simulink subsystem "RoboRio_Controls_sub"  (R2023b)
settings: Solver=VariableStepAuto  StartTime=0.0  StopTime=10.0  RelTol=1e-3
undefined symbols (not defined in the file): Odometry_IC_X, Odometry_IC_Y
libraries: Autonomous_lib x1, simulink_extras x1, Disabled_lib x1, Teleop_lib x1, Test_lib x1
settings Model: Creator=USER  LastModifiedBy=ander

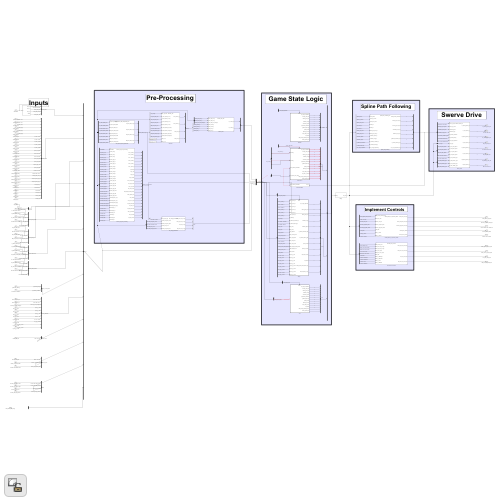
[thumbnail: Simulink's stored preview of the top-level diagram]
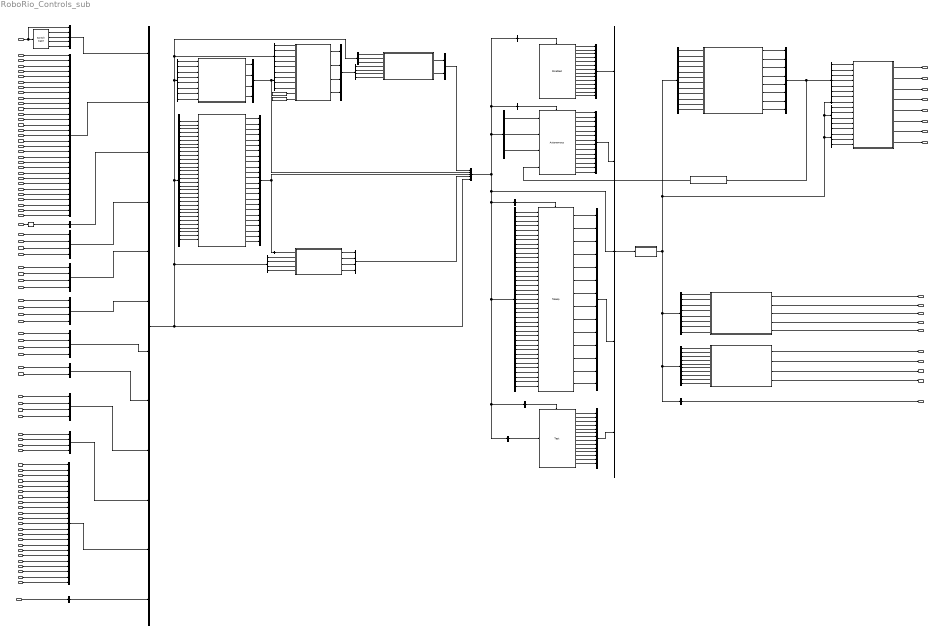
== system RoboRio_Controls_sub ==
  note: Game State Logic
  note: Swerve Drive
  note: Inputs
  note: Pre-Processing
  note: Spline Path
      | Following
  note: Implement Controls
  GameState : Inport
  Joystick_Left_X : Inport  Port=2
  Joystick_Left_Y : Inport  Port=3
  Joystick_Left_Z : Inport  Port=4
  Joystick_Right_X : Inport  Port=5
  Joystick_Right_Y : Inport  Port=6
  Joystick_Right_Z : Inport  Port=7
  Joystick_Left_B1 : Inport  Port=8
  Joystick_Left_B2 : Inport  Port=9
  Joystick_Left_B3 : Inport  Port=10
  Joystick_Left_B4 : Inport  Port=11
  Joystick_Left_B7 : Inport  Port=12
  Joystick_Left_B8 : Inport  Port=13
  Joystick_Left_B10 : Inport  Port=14
  Joystick_Right_B1 : Inport  Port=15
  Joystick_Right_B2 : Inport  Port=16
  Joystick_Right_B3 : Inport  Port=17
  Joystick_Right_B4 : Inport  Port=18
  Joystick_Right_POV : Inport  Port=19
  Joystick_Right_B7 : Inport  Port=20
  Joystick_Right_B8 : Inport  Port=21
  Joystick_Right_B10 : Inport  Port=22
  Gamepad_Stick_Left_X : Inport  Port=23
  Gamepad_Stick_Left_Y : Inport  Port=24
  Gamepad_Stick_Right_X : Inport  Port=25
  Gamepad_Stick_Right_Y : Inport  Port=26
  Gamepad_B1_A : Inport  Port=27
  Gamepad_B3_X : Inport  Port=28
  Gamepad_LB : Inport  Port=29
  Gamepad_LT : Inport  Port=30
  Gamepad_RB : Inport  Port=31
  Gamepad_RT : Inport  Port=32
  Gyro_Angle : Inport  Port=33
  FL_Drive_Motor_Speed : Inport  Port=34
  FR_Drive_Motor_Speed : Inport  Port=35
  BL_Drive_Motor_Speed : Inport  Port=36
  BR_Drive_Motor_Speed : Inport  Port=37
  FL_Drive_Motor_Rev : Inport  Port=38
  FR_Drive_Motor_Rev : Inport  Port=39
  BL_Drive_Motor_Rev : Inport  Port=40
  BR_Drive_Motor_Rev : Inport  Port=41
  FL_Steer_Module_Rev : Inport  Port=42
  FR_Steer_Module_Rev : Inport  Port=43
  BL_Steer_Module_Rev : Inport  Port=44
  BR_Steer_Module_Rev : Inport  Port=45
  FL_Steer_Module_Offset : Inport  Port=46
  FR_Steer_Module_Offset : Inport  Port=47
  BL_Steer_Module_Offset : Inport  Port=48
  BR_Steer_Module_Offset : Inport  Port=49
  Is_Absolute_Steering : Inport  Port=50
  Is_Absolute_Translation : Inport  Port=51
  Intake_TOF_Dist : Inport  Port=52
  Shooter_TOF_Dist : Inport  Port=53
  Shooter_Left_Motor_RPM : Inport  Port=54
  Shooter_Right_Motor_RPM : Inport  Port=55
  Encoder_Revs_Back_Lower : Inport  Port=56
  Encoder_Revs_Back_Upper : Inport  Port=57
  Encoder_Revs_Front : Inport  Port=58
  Encoder_Revs_Ball_Screw : Inport  Port=59
  Photon_Est_Pose_X : Inport  Port=60
  Photon_Est_Pose_Y : Inport  Port=61
  Photon_Est_Pose_Ambiguity : Inport  Port=62
  AT_Tag_4_Yaw : Inport  Port=63
  AT_Tag_5_Yaw : Inport  Port=64
  AT_Tag_6_Yaw : Inport  Port=65
  AT_Tag_7_Yaw : Inport  Port=66
  AT_Tag_11_Yaw : Inport  Port=67
  AT_Tag_12_Yaw : Inport  Port=68
  AT_Tag_13_Yaw : Inport  Port=69
  AT_Tag_14_Yaw : Inport  Port=70
  AT_Tag_15_Yaw : Inport  Port=71
  AT_Tag_16_Yaw : Inport  Port=72
  AT_Tag_4_Found : Inport  Port=73
  AT_Tag_5_Found : Inport  Port=74
  AT_Tag_6_Found : Inport  Port=75
  AT_Tag_7_Found : Inport  Port=76
  Line_Sensor_TOF_Range : Inport  Port=77
  AT_Tag_11_Found : Inport  Port=78
  AT_Tag_12_Found : Inport  Port=79
  AT_Tag_13_Found : Inport  Port=80
  AT_Tag_14_Found : Inport  Port=81
  AT_Tag_15_Found : Inport  Port=82
  AT_Tag_16_Found : Inport  Port=83
  Arm_Length_Calculation : Subsystem  ReferencedSubsystem=Arm_Length_Calculation
  Autonomous : Autonomous_lib/Autonomous  SystemSampleTime=-1  VariantActivationTime=update diagram  AllowFlexibleInterface=on  Latency=0  AutoFrameSizeCalculation=off
  Bus Creator : BusCreator  Inputs=5
  Bus Creator{1..2,4,12} (4 alike) : BusCreator  Inputs=14
  Bus Creator10 : BusCreator  Inputs=2
  Bus Creator11 : BusCreator  Inputs=12
  Bus Creator13 : BusCreator  Inputs=8
  Bus Creator{7..9,14..16,21..23} (9 alike) : BusCreator  Inputs=4
  Bus Creator17 : BusCreator  Inputs=5
  Bus Creator18 : BusCreator  Inputs=23
  Bus Creator19 : BusCreator  Inputs=2
  Bus Creator24 : BusCreator  Inputs=24
  Bus Creator25 : BusCreator  Inputs=1
  Bus Creator3 : BusCreator  Inputs=5
  Bus Creator5 : BusCreator  Inputs=31
  Bus Creator6 : BusCreator  Inputs=1
  Bus Selector : BusSelector  OutputSignals=Steering_Abs_Cmd_SPF,Steering_Rel_Cmd_SPF,Translation_Speed_SPF,Translation_Angle_SPF,Is_Absolute_Translation_SPF,Is_Absolute_Steering_SPF,Gyro_Angle_Adjustment_SPF
  Bus Selector1 : BusSelector  OutputSignals=Odom_Position_X,Odom_Position_Y,Odom_Delta_X,Odom_Delta_Y
  Bus Selector10 : BusSelector  OutputSignals=PreProcessing.Inputs.IMU_Sensor.Gyro_Angle
  Bus Selector11 : BusSelector  OutputSignals=State_Request_Arm,PreProcessing.Arms.Back_Lower_Arm_Length,PreProcessing.Arms.Back_Upper_Arm_Length,PreProcessing.Arms.Front_Arm_Length,PreProcessing.Arms.Ball_Screw_Arm_Length,Test_Mode,PreProcessing.Human_Inputs.Test_DC_BackUpper,PreProcessing.Human_Inputs.Test_DC_BackLower,PreProcessing.Human_Inputs.Test_DC_Front,PreProcessing.Human_Inputs.Test_DC_BallScrew
  Bus Selector12 : BusSelector  OutputSignals=Human_Inputs.Chain_Hook
  Bus Selector13 : BusSelector  OutputSignals=Game_States.GameState,Human_Inputs.Joystick_Left_X,Human_Inputs.Joystick_Left_Y,Human_Inputs.Joystick_Left_Z,Human_Inputs.Joystick_Right_X,Human_Inputs.Joystick_Right_Y,Human_Inputs.Joystick_Right_Z,Human_Inputs.Joystick_Left_B1,Human_Inputs.Joystick_Left_B2,Human_Inputs.Joystick_Left_B3,Human_Inputs.Joystick_Left_B4,Human_Inputs.Joystick_Left_B7,Human_Inputs.Joystick_Left_B8,Human_Inputs.Joystick_Left_B10,Human_Inputs.Joystick_Right_B1,Human_Inputs.Joystick_Right_B2,Human_Inputs.Joystick_Right_B3,Human_Inputs.Joystick_Right_B4,Human_Inputs.Joystick_Right_POV,Human_Inputs.Joystick_Right_B7,Human_Inputs.Joystick_Right_B8,Human_Inputs.Joystick_Right_B10,Human_Inputs.Gamepad_Stick_Left_X,Human_Inputs.Gamepad_Stick_Left_Y,Human_Inputs.Gamepad_Stick_Right_X,Human_Inputs.Gamepad_Stick_Right_Y,Human_Inputs.Gamepad_B1_A,Human_Inputs.Gamepad_B3_X,Human_Inputs.Gamepad_LB,Human_Inputs.Gamepad_LT,Human_Inputs.Gamepad_RB,Human_Inputs.Gamepad_RT
  Bus Selector14 : BusSelector  OutputSignals=Arm_Dist_Cal_Flag
  Bus Selector15 : BusSelector  OutputSignals=Chain_DutyCycle
  Bus Selector2 : BusSelector  OutputSignals=Inputs.Game_States.Game_State_Teleop
  Bus Selector3 : BusSelector  OutputSignals=Photon_Estimates.Photon_Est_Pose_X,Photon_Estimates.Photon_Est_Pose_Y,Photon_Estimates.Photon_Est_Pose_Ambiguity
  Bus Selector4 : BusSelector  OutputSignals=Inputs.Game_States.Game_State_Auto
  Bus Selector40 : BusSelector  OutputSignals=IMU_Sensor.Gyro_Angle,Drive_Motor_Revs.FL_Drive_Motor_Rev,Drive_Motor_Revs.FR_Drive_Motor_Rev,Drive_Motor_Revs.BL_Drive_Motor_Rev,Drive_Motor_Revs.BR_Drive_Motor_Rev
  Bus Selector41 : BusSelector  OutputSignals=Human_Inputs.Drive_Joystick_X,Human_Inputs.Drive_Joystick_Y,Human_Inputs.Drive_Joystick_Z,Human_Inputs.Steer_Joystick_X,Human_Inputs.Steer_Joystick_Y,Human_Inputs.Steer_Joystick_Z,Human_Inputs.Is_Boosting,Inputs.Motion_Control_Modes.Is_Absolute_Translation,Inputs.Motion_Control_Modes.Is_Absolute_Steering,Human_Inputs.Align_Trap,Human_Inputs.Align_Amp,Human_Inputs.Align_Speaker,Human_Inputs.Face_Toward_Driver,Human_Inputs.Face_Right_Driver,Human_Inputs.Face_Left_Driver,Human_Inputs.Face_Away_Driver,Human_Inputs.State_Request_Intake_Shooter,Human_Inputs.State_Request_Arm,Human_Inputs.Chain_Hook,Inputs.Photon_Estimates.AT_Tag_4_Yaw,Inputs.Photon_Estimates.AT_Tag_5_Yaw,Inputs.Photon_Estimates.AT_Tag_6_Yaw,Inputs.Photon_Estimates.AT_Tag_7_Yaw,Inputs.Photon_Estimates.AT_Tag_11_Yaw,Inputs.Photon_Estimates.AT_Tag_12_Yaw,Inputs.Photon_Estimates.AT_Tag_13_Yaw,Inputs.Photon_Estimates.AT_Tag_14_Yaw,Inputs.Photon_Estimates.AT_Tag_15_Yaw,Inputs.Photon_Estimates.AT_Tag_16_Yaw,Inputs.Photon_Estimates.AT_Tag_4_Found,Inputs.Photon_Estimates.AT_Tag_5_Found,Inputs.Photon_Estimates.AT_Tag_6_Found,Inputs.Photon_Estimates.AT_Tag_7_Found,Inputs.Photon_Estimates.AT_Tag_11_Found,Inputs.Photon_Estimates.AT_Tag_12_Found,Inputs.Photon_Estimates.AT_Tag_13_Found,Inputs.Photon_Estimates.AT_Tag_14_Found,Inputs.Photon_Estimates.AT_Tag_15_Found,Inputs.Photon_Estimates.AT_Tag_16_Found
  Bus Selector5 : BusSelector  OutputSignals=State_Request_Intake_Shooter,PreProcessing.Inputs.Intake_and_Shooter.Intake_TOF_Dist,PreProcessing.Inputs.Intake_and_Shooter.Shooter_TOF_Dist,PreProcessing.Inputs.Intake_and_Shooter.Shooter_Left_Motor_RPM,PreProcessing.Inputs.Intake_and_Shooter.Shooter_Right_Motor_RPM,Test_Mode,PreProcessing.Human_Inputs.Test_DC_Intake,PreProcessing.Human_Inputs.Test_DC_Shooter
  Bus Selector50 : BusSelector  OutputSignals=PreProcessing.Inputs.Drive_Motor_Speeds.FL_Drive_Motor_Speed,PreProcessing.Inputs.Drive_Motor_Speeds.FR_Drive_Motor_Speed,PreProcessing.Inputs.Drive_Motor_Speeds.BL_Drive_Motor_Speed,PreProcessing.Inputs.Drive_Motor_Speeds.BR_Drive_Motor_Speed
  Bus Selector52 : BusSelector  OutputSignals=PreProcessing.Steer_Module_Angles.FL_Steer_Module_Angle,PreProcessing.Steer_Module_Angles.FR_Steer_Module_Angle,PreProcessing.Steer_Module_Angles.BL_Steer_Module_Angle,PreProcessing.Steer_Module_Angles.BR_Steer_Module_Angle
  Bus Selector57 : BusSelector  OutputSignals=Steer_Module_Revs.FL_Steer_Module_Rev,Steer_Module_Offsets.FL_Steer_Module_Offset,Steer_Module_Revs.FR_Steer_Module_Rev,Steer_Module_Offsets.FR_Steer_Module_Offset,Steer_Module_Revs.BL_Steer_Module_Rev,Steer_Module_Offsets.BL_Steer_Module_Offset,Steer_Module_Revs.BR_Steer_Module_Rev,Steer_Module_Offsets.BR_Steer_Module_Offset
  Bus Selector58 : BusSelector  OutputSignals=FL_Steer_Module_Angle,FR_Steer_Module_Angle,BL_Steer_Module_Angle,BR_Steer_Module_Angle
  Bus Selector59 : BusSelector  OutputSignals=EKF.KF_Position_X,EKF.KF_Position_Y,Inputs.Autonomous.Line_Sensor_TOF_Range
  Bus Selector6 : BusSelector  OutputSignals=Inputs.Game_States.Game_State_Disabled
  Bus Selector7 : BusSelector  OutputSignals=Arms.Encoder_Revs_Back_Lower,Arms.Encoder_Revs_Back_Upper,Arms.Encoder_Revs_Front,Arms.Encoder_Revs_Ball_Screw
  Bus Selector8 : BusSelector  OutputSignals=Inputs.Game_States.Game_State_Test
  Bus Selector9 : BusSelector  OutputSignals=Spline_Enable,Spline_Ref_Poses,Spline_Num_Poses,PreProcessing.EKF.KF_Position_X,PreProcessing.EKF.KF_Position_Y,Steering_Abs_Cmd,Steering_Rel_Cmd,Translation_Speed,Translation_Angle,Is_Absolute_Translation,Is_Absolute_Steering,Gyro_Angle_Adjustment
  Constant : Constant  Value=Odometry_IC_X
  Constant1 : Constant  Value=Odometry_IC_Y
  Degrees to Radians : simulink_extras/Transformations/Degrees to Radians
  Disabled : Disabled_lib/Disabled  SystemSampleTime=-1  VariantActivationTime=update diagram  AllowFlexibleInterface=on  Latency=0  AutoFrameSizeCalculation=off
  Human_Input_Pre_Processing : Subsystem  ReferencedSubsystem=Human_Input_Pre_Processing
  Intake_Rollers_and_Shooter_Wheels : Subsystem  ReferencedSubsystem=Intake_Rollers_and_Shooter_Wheels
  Internal Feedback : Subsystem
  Kalman_Filter : Subsystem  ReferencedSubsystem=Kalman_Filter_sub
  Merge : Subsystem
  Odometry : Subsystem  ReferencedSubsystem=Odometry_sub
  Shooter_Arm_Controls : Subsystem  ReferencedSubsystem=Shooter_Arm_Controls
  Spline_Path_Following : Subsystem  ReferencedSubsystem=Spline_Path_Following_sub
  Steer_Module_Offset_Adjustments : Subsystem  ReferencedSubsystem=Steer_Module_Offset_Adjustments_sub
  Swerve_Drive : Subsystem  ReferencedSubsystem=Swerve_Drive_sub
  Switch Case : SwitchCase  CaseConditions={0,1,2}
  Teleop : Teleop_lib/Teleop  SystemSampleTime=-1  VariantActivationTime=update diagram  AllowFlexibleInterface=on  Latency=0  AutoFrameSizeCalculation=off
  Test : Test_lib/Test  SystemSampleTime=-1  VariantActivationTime=update diagram  AllowFlexibleInterface=on  Latency=0  AutoFrameSizeCalculation=off
  FL_Drive_Motor_DC : Outport
  FL_Steering_Motor_DC : Outport  Port=2
  FR_Drive_Motor_DC : Outport  Port=3
  BL_Drive_Motor_DC : Outport  Port=4
  FR_Steering_Motor_DC : Outport  Port=5
  BL_Steering_Motor_DC : Outport  Port=6
  BR_Drive_Motor_DC : Outport  Port=7
  BR_Steering_Motor_DC : Outport  Port=8
  Intake_Motor_DutyCycle : Outport  Port=9
  Shooter_Left_Motor_DutyCycle : Outport  Port=10
  Shooter_Right_Motor_DutyCycle : Outport  Port=11
  Shooter_Brake_Enable : Outport  Port=12
  Back_Upper_Arm_DutyCycle : Outport  Port=13
  Shooter_Servo_Position : Outport  Port=14
  Back_Lower_Arm_DutyCycle : Outport  Port=15
  Front_Arm_DutyCycle : Outport  Port=16
  Ball_Screw_Arm_DutyCycle : Outport  Port=17
  Chain_DutyCycle : Outport  Port=18
  wires:
  Teleop/1 -> Bus Creator2/1
  Teleop/2 -> Bus Creator2/2
  Teleop/3 -> Bus Creator2/3
  Teleop/4 -> Bus Creator2/4
  Teleop/5 -> Bus Creator2/5
  Bus Creator4/1 -> Bus Creator3/1  "Disabled"
  Bus Creator1/1 -> Bus Creator3/2  "Autonomous"
  Bus Creator2/1 -> Bus Creator3/4  "Teleop"
  Switch Case/1 -> Bus Creator/2  "Game_State_Disabled"
  Switch Case/2 -> Bus Creator/3  "Game_State_Auto"
  Switch Case/3 -> Bus Creator/4  "Game_State_Teleop"
  GameState/1 -> Bus Creator/1, Switch Case/1  "GameState"
  Bus Creator12/1 -> Bus Creator3/5  "Test"
  Switch Case/4 -> Bus Creator/5  "Game_State_Test"
  Gyro_Angle/1 -> Degrees to Radians/1
  Bus Creator5/1 -> Bus Creator11/2  "Human_Inputs"
  Bus Creator6/1 -> Bus Creator11/3  "IMU_Sensor"
  FL_Drive_Motor_Speed/1 -> Bus Creator7/1  "FL_Drive_Motor_Speed"
  FR_Drive_Motor_Speed/1 -> Bus Creator7/2  "FR_Drive_Motor_Speed"
  BL_Drive_Motor_Speed/1 -> Bus Creator7/3  "BL_Drive_Motor_Speed"
  BR_Drive_Motor_Speed/1 -> Bus Creator7/4  "BR_Drive_Motor_Speed"
  FL_Steer_Module_Rev/1 -> Bus Creator8/1  "FL_Steer_Module_Rev"
  BL_Steer_Module_Rev/1 -> Bus Creator8/3  "BL_Steer_Module_Rev"
  BR_Steer_Module_Rev/1 -> Bus Creator8/4  "BR_Steer_Module_Rev"
  FR_Steer_Module_Rev/1 -> Bus Creator8/2  "FR_Steer_Module_Rev"
  Bus Creator7/1 -> Bus Creator11/4  "Drive_Motor_Speeds"
  Bus Creator8/1 -> Bus Creator11/6  "Steer_Module_Revs"
  FL_Steer_Module_Offset/1 -> Bus Creator9/1  "FL_Steer_Module_Offset"
  FR_Steer_Module_Offset/1 -> Bus Creator9/2  "FR_Steer_Module_Offset"
  BL_Steer_Module_Offset/1 -> Bus Creator9/3  "BL_Steer_Module_Offset"
  BR_Steer_Module_Offset/1 -> Bus Creator9/4  "BR_Steer_Module_Offset"
  Bus Creator9/1 -> Bus Creator11/7  "Steer_Module_Offsets"
  Is_Absolute_Steering/1 -> Bus Creator10/1  "Is_Absolute_Steering"
  Is_Absolute_Translation/1 -> Bus Creator10/2  "Is_Absolute_Translation"
  Bus Creator10/1 -> Bus Creator11/8  "Motion_Control_Modes"
  Teleop/6 -> Bus Creator2/6
  Teleop/7 -> Bus Creator2/7
  Autonomous/2 -> Bus Creator1/2
  Autonomous/4 -> Bus Creator1/4
  Autonomous/1 -> Bus Creator1/1
  Autonomous/5 -> Bus Creator1/5
  Autonomous/7 -> Bus Creator1/7
  Autonomous/3 -> Bus Creator1/3
  Autonomous/6 -> Bus Creator1/6
  Disabled/2 -> Bus Creator4/2
  Disabled/4 -> Bus Creator4/4
  Disabled/1 -> Bus Creator4/1
  Disabled/5 -> Bus Creator4/5
  Disabled/7 -> Bus Creator4/7
  Disabled/3 -> Bus Creator4/3
  Disabled/6 -> Bus Creator4/6
  Test/2 -> Bus Creator12/2
  Test/4 -> Bus Creator12/4
  Test/1 -> Bus Creator12/1
  Test/5 -> Bus Creator12/5
  Test/7 -> Bus Creator12/7
  Test/3 -> Bus Creator12/3
  Test/6 -> Bus Creator12/6
  Bus Creator/1 -> Bus Creator11/1  "Game_States"
  Bus Selector2/1 -> Teleop/Action  "<Game_State_Teleop>"
  Bus Selector4/1 -> Autonomous/Action  "<Game_State_Auto>"
  Bus Selector6/1 -> Disabled/Action  "<Game_State_Disabled>"
  Bus Selector8/1 -> Test/Action  "<Game_State_Test>"
  Bus Selector50/4 -> Swerve_Drive/12  "<BR_Drive_Motor_Speed>"
  Bus Selector50/3 -> Swerve_Drive/11  "<BL_Drive_Motor_Speed>"
  Bus Selector50/2 -> Swerve_Drive/10  "<FR_Drive_Motor_Speed>"
  Bus Selector50/1 -> Swerve_Drive/9  "<FL_Drive_Motor_Speed>"
  Swerve_Drive/1 -> FL_Steering_Motor_DC/1
  Swerve_Drive/2 -> FL_Drive_Motor_DC/1
  Swerve_Drive/3 -> FR_Steering_Motor_DC/1
  Swerve_Drive/4 -> FR_Drive_Motor_DC/1
  Swerve_Drive/5 -> BL_Steering_Motor_DC/1
  Swerve_Drive/6 -> BL_Drive_Motor_DC/1
  Swerve_Drive/7 -> BR_Steering_Motor_DC/1
  Swerve_Drive/8 -> BR_Drive_Motor_DC/1
  Joystick_Left_B1/1 -> Bus Creator5/7  "Joystick_Left_B1"
  Bus Creator14/1 -> Bus Creator11/5  "Drive_Motor_Revs"
  FL_Drive_Motor_Rev/1 -> Bus Creator14/1  "FL_Drive_Motor_Rev"
  FR_Drive_Motor_Rev/1 -> Bus Creator14/2  "FR_Drive_Motor_Rev"
  BL_Drive_Motor_Rev/1 -> Bus Creator14/3  "BL_Drive_Motor_Rev"
  BR_Drive_Motor_Rev/1 -> Bus Creator14/4  "BR_Drive_Motor_Rev"
  Bus Selector40/2 -> Odometry/2  "<FL_Drive_Motor_Rev>"
  Bus Selector40/3 -> Odometry/3  "<FR_Drive_Motor_Rev>"
  Bus Selector40/4 -> Odometry/4  "<BL_Drive_Motor_Rev>"
  Bus Selector40/5 -> Odometry/5  "<BR_Drive_Motor_Rev>"
  Bus Selector40/1 -> Odometry/1  "<Gyro_Angle>"
  Constant1/1 -> Odometry/11
  Constant/1 -> Odometry/10
  Bus Selector57/1 -> Steer_Module_Offset_Adjustments/1  "<FL_Steer_Module_Rev>"
  Bus Selector57/2 -> Steer_Module_Offset_Adjustments/2  "<FL_Steer_Module_Offset>"
  Bus Selector57/3 -> Steer_Module_Offset_Adjustments/3  "<FR_Steer_Module_Rev>"
  Bus Selector57/4 -> Steer_Module_Offset_Adjustments/4  "<FR_Steer_Module_Offset>"
  Bus Selector57/5 -> Steer_Module_Offset_Adjustments/5  "<BL_Steer_Module_Rev>"
  Bus Selector57/6 -> Steer_Module_Offset_Adjustments/6  "<BL_Steer_Module_Offset>"
  Bus Selector57/7 -> Steer_Module_Offset_Adjustments/7  "<BR_Steer_Module_Rev>"
  Bus Selector57/8 -> Steer_Module_Offset_Adjustments/8  "<BR_Steer_Module_Offset>"
  Steer_Module_Offset_Adjustments/2 -> Bus Creator15/2
  Steer_Module_Offset_Adjustments/1 -> Bus Creator15/1
  Steer_Module_Offset_Adjustments/3 -> Bus Creator15/3
  Steer_Module_Offset_Adjustments/4 -> Bus Creator15/4
  Bus Creator15/1 -> Bus Creator17/2, Bus Selector58/1  "Steer_Module_Angles"
  Bus Selector58/1 -> Odometry/6  "<FL_Steer_Module_Angle>"
  Bus Selector58/2 -> Odometry/7  "<FR_Steer_Module_Angle>"
  Bus Selector58/3 -> Odometry/8  "<BL_Steer_Module_Angle>"
  Bus Selector58/4 -> Odometry/9  "<BR_Steer_Module_Angle>"
  Bus Creator16/1 -> Bus Selector1/1  "Odometry"
  Bus Creator11/1 -> Bus Creator17/5, Bus Selector7/1, Bus Selector13/1, Bus Selector57/1, Bus Selector40/1, Bus Selector3/1  "Inputs"
  Bus Selector52/1 -> Swerve_Drive/13  "<FL_Steer_Module_Angle>"
  Bus Selector52/2 -> Swerve_Drive/14  "<FR_Steer_Module_Angle>"
  Bus Selector52/3 -> Swerve_Drive/15  "<BL_Steer_Module_Angle>"
  Bus Selector52/4 -> Swerve_Drive/16  "<BR_Steer_Module_Angle>"
  Degrees to Radians/1 -> Bus Creator6/1  "Gyro_Angle"
  Disabled/8 -> Bus Creator4/8
  Disabled/9 -> Bus Creator4/9
  Disabled/10 -> Bus Creator4/10
  Autonomous/8 -> Bus Creator1/8
  Autonomous/9 -> Bus Creator1/9
  Autonomous/10 -> Bus Creator1/10
  Teleop/8 -> Bus Creator2/8
  Teleop/9 -> Bus Creator2/9
  Teleop/10 -> Bus Creator2/10
  Test/8 -> Bus Creator12/8
  Test/9 -> Bus Creator12/9
  Test/10 -> Bus Creator12/10
  Merge/1(Bus_Out) -> Bus Selector5/1, Bus Selector11/1, Bus Selector15/1, Bus Selector52/1, Bus Selector50/1, Bus Selector10/1, Bus Selector9/1
  Bus Creator3/1 -> Merge/1(Bus_In)
  Bus Selector10/1 -> Swerve_Drive/8  "<Gyro_Angle>"
  Bus Selector59/1 -> Autonomous/1  "<KF_Position_X>"
  Bus Selector59/2 -> Autonomous/2  "<KF_Position_Y>"
  Bus Selector41/9 -> Teleop/9  "<Is_Absolute_Steering>"
  Bus Selector41/8 -> Teleop/8  "<Is_Absolute_Translation>"
  Bus Selector9/1 -> Spline_Path_Following/1  "<Spline_Enable>"
  Bus Selector9/2 -> Spline_Path_Following/2  "<Spline_Ref_Poses>"
  Bus Selector9/3 -> Spline_Path_Following/3  "<Spline_Num_Poses>"
  Bus Selector9/6 -> Spline_Path_Following/6  "<Steering_Abs_Cmd>"
  Bus Selector9/7 -> Spline_Path_Following/7  "<Steering_Rel_Cmd>"
  Bus Selector9/8 -> Spline_Path_Following/8  "<Translation_Speed>"
  Bus Selector9/9 -> Spline_Path_Following/9  "<Translation_Angle>"
  Bus Selector9/10 -> Spline_Path_Following/10  "<Is_Absolute_Translation>"
  Bus Selector9/11 -> Spline_Path_Following/11  "<Is_Absolute_Steering>"
  Bus Selector9/12 -> Spline_Path_Following/12  "<Gyro_Angle_Adjustment>"
  Spline_Path_Following/2 -> Bus Creator13/2
  Spline_Path_Following/3 -> Bus Creator13/3
  Spline_Path_Following/4 -> Bus Creator13/4
  Spline_Path_Following/5 -> Bus Creator13/5
  Spline_Path_Following/6 -> Bus Creator13/6
  Spline_Path_Following/7 -> Bus Creator13/7
  Spline_Path_Following/8 -> Bus Creator13/8
  Bus Creator13/1 -> Internal Feedback/1(Bus_In), Bus Selector/1
  Bus Selector/5 -> Swerve_Drive/5  "<Is_Absolute_Translation_SPF>"
  Bus Selector/4 -> Swerve_Drive/4  "<Translation_Angle_SPF>"
  Bus Selector/6 -> Swerve_Drive/6  "<Is_Absolute_Steering_SPF>"
  Bus Selector/3 -> Swerve_Drive/3  "<Translation_Speed_SPF>"
  Bus Selector/7 -> Swerve_Drive/7  "<Gyro_Angle_Adjustment_SPF>"
  Bus Selector/2 -> Swerve_Drive/2  "<Steering_Rel_Cmd_SPF>"
  Bus Selector/1 -> Swerve_Drive/1  "<Steering_Abs_Cmd_SPF>"
  Spline_Path_Following/1 -> Bus Creator13/1
  Photon_Est_Pose_X/1 -> Bus Creator18/1  "Photon_Est_Pose_X"
  Photon_Est_Pose_Y/1 -> Bus Creator18/2  "Photon_Est_Pose_Y"
  Photon_Est_Pose_Ambiguity/1 -> Bus Creator18/3  "Photon_Est_Pose_Ambiguity"
  Bus Selector1/3 -> Kalman_Filter/6  "<Odom_Delta_X>"
  Bus Selector1/4 -> Kalman_Filter/7  "<Odom_Delta_Y>"
  Bus Selector3/3 -> Kalman_Filter/3  "<Photon_Est_Pose_Ambiguity>"
  Bus Selector3/2 -> Kalman_Filter/2  "<Photon_Est_Pose_Y>"
  Bus Selector3/1 -> Kalman_Filter/1  "<Photon_Est_Pose_X>"
  Kalman_Filter/1 -> Bus Creator19/1
  Kalman_Filter/2 -> Bus Creator19/2
  Bus Selector9/4 -> Spline_Path_Following/4  "<KF_Position_X>"
  Bus Selector9/5 -> Spline_Path_Following/5  "<KF_Position_Y>"
  Bus Creator19/1 -> Bus Creator17/1  "EKF"
  Odometry/1 -> Bus Creator16/1
  Odometry/2 -> Bus Creator16/2
  Odometry/3 -> Bus Creator16/3
  Odometry/4 -> Bus Creator16/4
  Bus Selector1/2 -> Kalman_Filter/5  "<Odom_Position_Y>"
  Bus Selector1/1 -> Kalman_Filter/4  "<Odom_Position_X>"
  Bus Selector5/2 -> Intake_Rollers_and_Shooter_Wheels/2  "<Intake_TOF_Dist>"
  Intake_Rollers_and_Shooter_Wheels/1 -> Intake_Motor_DutyCycle/1
  Shooter_TOF_Dist/1 -> Bus Creator21/2  "Shooter_TOF_Dist"
  Shooter_Left_Motor_RPM/1 -> Bus Creator21/3  "Shooter_Left_Motor_RPM"
  Shooter_Right_Motor_RPM/1 -> Bus Creator21/4  "Shooter_Right_Motor_RPM"
  Bus Selector5/3 -> Intake_Rollers_and_Shooter_Wheels/3  "<Shooter_TOF_Dist>"
  Bus Selector5/4 -> Intake_Rollers_and_Shooter_Wheels/4  "<Shooter_Left_Motor_RPM>"
  Bus Selector5/5 -> Intake_Rollers_and_Shooter_Wheels/5  "<Shooter_Right_Motor_RPM>"
  Intake_Rollers_and_Shooter_Wheels/2 -> Shooter_Left_Motor_DutyCycle/1
  Intake_Rollers_and_Shooter_Wheels/3 -> Shooter_Right_Motor_DutyCycle/1
  Intake_Rollers_and_Shooter_Wheels/4 -> Shooter_Brake_Enable/1
  Intake_Rollers_and_Shooter_Wheels/5 -> Shooter_Servo_Position/1
  Encoder_Revs_Back_Lower/1 -> Bus Creator22/1  "Encoder_Revs_Back_Lower"
  Encoder_Revs_Back_Upper/1 -> Bus Creator22/2  "Encoder_Revs_Back_Upper"
  Encoder_Revs_Front/1 -> Bus Creator22/3  "Encoder_Revs_Front"
  Encoder_Revs_Ball_Screw/1 -> Bus Creator22/4  "Encoder_Revs_Ball_Screw"
  Arm_Length_Calculation/1 -> Bus Creator23/1
  Arm_Length_Calculation/2 -> Bus Creator23/2
  Arm_Length_Calculation/3 -> Bus Creator23/3
  Arm_Length_Calculation/4 -> Bus Creator23/4
  Bus Creator23/1 -> Bus Creator17/4  "Arms"
  Bus Selector11/2 -> Shooter_Arm_Controls/2  "<Back_Lower_Arm_Length>"
  Bus Selector11/3 -> Shooter_Arm_Controls/3  "<Back_Upper_Arm_Length>"
  Bus Selector11/4 -> Shooter_Arm_Controls/4  "<Front_Arm_Length>"
  Bus Selector11/5 -> Shooter_Arm_Controls/5  "<Ball_Screw_Arm_Length>"
  Shooter_Arm_Controls/1 -> Back_Upper_Arm_DutyCycle/1
  Shooter_Arm_Controls/2 -> Back_Lower_Arm_DutyCycle/1
  Shooter_Arm_Controls/3 -> Front_Arm_DutyCycle/1
  Shooter_Arm_Controls/4 -> Ball_Screw_Arm_DutyCycle/1
  Bus Selector7/1 -> Arm_Length_Calculation/2  "<Encoder_Revs_Back_Lower>"
  Bus Selector7/2 -> Arm_Length_Calculation/3  "<Encoder_Revs_Back_Upper>"
  Bus Selector7/3 -> Arm_Length_Calculation/4  "<Encoder_Revs_Front>"
  Bus Selector7/4 -> Arm_Length_Calculation/5  "<Encoder_Revs_Ball_Screw>"
  Test/11 -> Bus Creator12/11
  Teleop/11 -> Bus Creator2/11
  Autonomous/11 -> Bus Creator1/11
  Disabled/11 -> Bus Creator4/11
  Joystick_Right_B4/1 -> Bus Creator5/17  "Joystick_Right_B4"
  Joystick_Right_B3/1 -> Bus Creator5/16  "Joystick_Right_B3"
  Joystick_Right_B2/1 -> Bus Creator5/15  "Joystick_Right_B2"
  Joystick_Right_B1/1 -> Bus Creator5/14  "Joystick_Right_B1"
  Joystick_Left_B10/1 -> Bus Creator5/13  "Joystick_Left_B10"
  Joystick_Left_B8/1 -> Bus Creator5/12  "Joystick_Left_B8"
  Joystick_Left_B4/1 -> Bus Creator5/10  "Joystick_Left_B4"
  Joystick_Left_B3/1 -> Bus Creator5/9  "Joystick_Left_B3"
  Joystick_Left_B2/1 -> Bus Creator5/8  "Joystick_Left_B2"
  Bus Selector13/5 -> Human_Input_Pre_Processing/5  "<Joystick_Right_X>"
  Bus Selector13/6 -> Human_Input_Pre_Processing/6  "<Joystick_Right_Y>"
  Bus Selector13/2 -> Human_Input_Pre_Processing/2  "<Joystick_Left_X>"
  Bus Selector13/4 -> Human_Input_Pre_Processing/4  "<Joystick_Left_Z>"
  Bus Selector13/3 -> Human_Input_Pre_Processing/3  "<Joystick_Left_Y>"
  Bus Selector13/7 -> Human_Input_Pre_Processing/7  "<Joystick_Right_Z>"
  Bus Selector13/8 -> Human_Input_Pre_Processing/8  "<Joystick_Left_B1>"
  Bus Selector13/9 -> Human_Input_Pre_Processing/9  "<Joystick_Left_B2>"
  Bus Selector13/10 -> Human_Input_Pre_Processing/10  "<Joystick_Left_B3>"
  Bus Selector13/11 -> Human_Input_Pre_Processing/11  "<Joystick_Left_B4>"
  Bus Selector13/13 -> Human_Input_Pre_Processing/13  "<Joystick_Left_B8>"
  Bus Selector13/14 -> Human_Input_Pre_Processing/14  "<Joystick_Left_B10>"
  Bus Selector13/15 -> Human_Input_Pre_Processing/15  "<Joystick_Right_B1>"
  Bus Selector13/16 -> Human_Input_Pre_Processing/16  "<Joystick_Right_B2>"
  Bus Selector13/17 -> Human_Input_Pre_Processing/17  "<Joystick_Right_B3>"
  Bus Selector13/18 -> Human_Input_Pre_Processing/18  "<Joystick_Right_B4>"
  Bus Selector13/21 -> Human_Input_Pre_Processing/21  "<Joystick_Right_B8>"
  Bus Selector13/22 -> Human_Input_Pre_Processing/22  "<Joystick_Right_B10>"
  Bus Selector13/24 -> Human_Input_Pre_Processing/24  "<Gamepad_Stick_Left_Y>"
  Bus Selector13/26 -> Human_Input_Pre_Processing/26  "<Gamepad_Stick_Right_Y>"
  Bus Selector13/27 -> Human_Input_Pre_Processing/27  "<Gamepad_B1_A>"
  Bus Selector13/29 -> Human_Input_Pre_Processing/29  "<Gamepad_LB>"
  Bus Selector13/30 -> Human_Input_Pre_Processing/30  "<Gamepad_LT>"
  Bus Selector13/31 -> Human_Input_Pre_Processing/31  "<Gamepad_RB>"
  Bus Selector13/32 -> Human_Input_Pre_Processing/32  "<Gamepad_RT>"
  Joystick_Left_Y/1 -> Bus Creator5/2  "Joystick_Left_Y"
  Joystick_Left_X/1 -> Bus Creator5/1  "Joystick_Left_X"
  Joystick_Left_Z/1 -> Bus Creator5/3  "Joystick_Left_Z"
  Joystick_Right_X/1 -> Bus Creator5/4  "Joystick_Right_X"
  Joystick_Right_Y/1 -> Bus Creator5/5  "Joystick_Right_Y"
  Joystick_Right_Z/1 -> Bus Creator5/6  "Joystick_Right_Z"
  Gamepad_Stick_Left_Y/1 -> Bus Creator5/23  "Gamepad_Stick_Left_Y"
  Joystick_Right_B10/1 -> Bus Creator5/21  "Joystick_Right_B10"
  Gamepad_Stick_Right_Y/1 -> Bus Creator5/25  "Gamepad_Stick_Right_Y"
  Joystick_Right_B8/1 -> Bus Creator5/20  "Joystick_Right_B8"
  Gamepad_B1_A/1 -> Bus Creator5/26  "Gamepad_B1_A"
  Joystick_Right_POV/1 -> Bus Creator5/18  "Joystick_Right_POV"
  Gamepad_LB/1 -> Bus Creator5/28  "Gamepad_LB"
  Gamepad_LT/1 -> Bus Creator5/29  "Gamepad_LT"
  Gamepad_RB/1 -> Bus Creator5/30  "Gamepad_RB"
  Gamepad_RT/1 -> Bus Creator5/31  "Gamepad_RT"
  Bus Selector13/19 -> Human_Input_Pre_Processing/19  "<Joystick_Right_POV>"
  Human_Input_Pre_Processing/1 -> Bus Creator24/1
  Human_Input_Pre_Processing/2 -> Bus Creator24/2
  Human_Input_Pre_Processing/3 -> Bus Creator24/3
  Human_Input_Pre_Processing/4 -> Bus Creator24/4
  Human_Input_Pre_Processing/5 -> Bus Creator24/5
  Human_Input_Pre_Processing/6 -> Bus Creator24/6
  Human_Input_Pre_Processing/7 -> Bus Creator24/7
  Human_Input_Pre_Processing/8 -> Bus Creator24/8
  Human_Input_Pre_Processing/9 -> Bus Creator24/9
  Human_Input_Pre_Processing/10 -> Bus Creator24/10
  Human_Input_Pre_Processing/11 -> Bus Creator24/11
  Human_Input_Pre_Processing/12 -> Bus Creator24/12
  Human_Input_Pre_Processing/13 -> Bus Creator24/13
  Human_Input_Pre_Processing/14 -> Bus Creator24/14
  Human_Input_Pre_Processing/15 -> Bus Creator24/15
  Human_Input_Pre_Processing/16 -> Bus Creator24/16
  Bus Creator24/1 -> Bus Creator17/3, Bus Selector14/1  "Human_Inputs"
  Bus Selector41/1 -> Teleop/1  "<Drive_Joystick_X>"
  Bus Selector41/2 -> Teleop/2  "<Drive_Joystick_Y>"
  Bus Selector41/3 -> Teleop/3  "<Drive_Joystick_Z>"
  Bus Selector41/4 -> Teleop/4  "<Steer_Joystick_X>"
  Bus Selector41/5 -> Teleop/5  "<Steer_Joystick_Y>"
  Bus Selector41/6 -> Teleop/6  "<Steer_Joystick_Z>"
  Bus Selector41/7 -> Teleop/7  "<Is_Boosting>"
  Gamepad_B3_X/1 -> Bus Creator5/27  "Gamepad_B3_X"
  Bus Selector13/28 -> Human_Input_Pre_Processing/28  "<Gamepad_B3_X>"
  Human_Input_Pre_Processing/18 -> Bus Creator24/18
  Bus Selector14/1 -> Arm_Length_Calculation/1  "<Arm_Dist_Cal_Flag>"
  Disabled/12 -> Bus Creator4/12
  Disabled/13 -> Bus Creator4/13
  Autonomous/12 -> Bus Creator1/12
  Autonomous/13 -> Bus Creator1/13
  Teleop/12 -> Bus Creator2/12
  Teleop/13 -> Bus Creator2/13
  Test/12 -> Bus Creator12/12
  Test/13 -> Bus Creator12/13
  Bus Selector41/10 -> Teleop/10  "<Align_Trap>"
  Bus Selector41/11 -> Teleop/11  "<Align_Amp>"
  Bus Selector41/12 -> Teleop/12  "<Align_Speaker>"
  Bus Selector41/13 -> Teleop/13  "<Face_Toward_Driver>"
  Bus Selector41/14 -> Teleop/14  "<Face_Right_Driver>"
  Bus Selector41/15 -> Teleop/15  "<Face_Left_Driver>"
  Bus Selector41/16 -> Teleop/16  "<Face_Away_Driver>"
  Bus Selector41/17 -> Teleop/17  "<State_Request_Intake_Shooter>"
  Bus Selector41/18 -> Teleop/18  "<State_Request_Arm>"
  Bus Selector11/1 -> Shooter_Arm_Controls/1  "<State_Request_Arm>"
  Bus Selector5/1 -> Intake_Rollers_and_Shooter_Wheels/1  "<State_Request_Intake_Shooter>"
  AT_Tag_4_Yaw/1 -> Bus Creator18/4  "AT_Tag_4_Yaw"
  AT_Tag_5_Yaw/1 -> Bus Creator18/5  "AT_Tag_5_Yaw"
  AT_Tag_6_Yaw/1 -> Bus Creator18/6  "AT_Tag_6_Yaw"
  AT_Tag_7_Yaw/1 -> Bus Creator18/7  "AT_Tag_7_Yaw"
  Bus Selector13/1 -> Human_Input_Pre_Processing/1  "<GameState>"
  Bus Selector11/6 -> Shooter_Arm_Controls/6  "<Test_Mode>"
  Human_Input_Pre_Processing/19 -> Bus Creator24/19
  Human_Input_Pre_Processing/20 -> Bus Creator24/20
  Human_Input_Pre_Processing/21 -> Bus Creator24/21
  Human_Input_Pre_Processing/22 -> Bus Creator24/22
  Human_Input_Pre_Processing/23 -> Bus Creator24/23
  Human_Input_Pre_Processing/24 -> Bus Creator24/24
  Bus Selector11/8 -> Shooter_Arm_Controls/8  "<Test_DC_BackLower>"
  Bus Selector11/7 -> Shooter_Arm_Controls/7  "<Test_DC_BackUpper>"
  Bus Selector11/9 -> Shooter_Arm_Controls/9  "<Test_DC_Front>"
  Bus Selector11/10 -> Shooter_Arm_Controls/10  "<Test_DC_BallScrew>"
  Bus Selector5/6 -> Intake_Rollers_and_Shooter_Wheels/6  "<Test_Mode>"
  Bus Selector5/7 -> Intake_Rollers_and_Shooter_Wheels/7  "<Test_DC_Intake>"
  Bus Selector5/8 -> Intake_Rollers_and_Shooter_Wheels/8  "<Test_DC_Shooter>"
  Gamepad_Stick_Left_X/1 -> Bus Creator5/22  "Gamepad_Stick_Left_X"
  Gamepad_Stick_Right_X/1 -> Bus Creator5/24  "Gamepad_Stick_Right_X"
  Bus Selector13/23 -> Human_Input_Pre_Processing/23  "<Gamepad_Stick_Left_X>"
  Bus Selector13/25 -> Human_Input_Pre_Processing/25  "<Gamepad_Stick_Right_X>"
  Bus Creator17/1 -> Bus Selector59/1, Bus Selector4/1, Bus Selector6/1, Bus Creator3/3, Bus Selector2/1, Bus Selector41/1, Bus Selector12/1, Bus Selector8/1  "PreProcessing"
  Intake_TOF_Dist/1 -> Bus Creator21/1  "Intake_TOF_Dist"
  Line_Sensor_TOF_Range/1 -> Bus Creator25/1  "Line_Sensor_TOF_Range"
  Bus Creator21/1 -> Bus Creator11/9  "Intake_and_Shooter"
  Bus Creator22/1 -> Bus Creator11/10  "Arms"
  Bus Creator18/1 -> Bus Creator11/11  "Photon_Estimates"
  Bus Creator25/1 -> Bus Creator11/12  "Autonomous"
  Internal Feedback/1(Robot_Reached_Destination) -> Autonomous/4
  Bus Selector59/3 -> Autonomous/3  "<Line_Sensor_TOF_Range>"
  AT_Tag_11_Yaw/1 -> Bus Creator18/8  "AT_Tag_11_Yaw"
  AT_Tag_12_Yaw/1 -> Bus Creator18/9  "AT_Tag_12_Yaw"
  AT_Tag_13_Yaw/1 -> Bus Creator18/10  "AT_Tag_13_Yaw"
  AT_Tag_14_Yaw/1 -> Bus Creator18/11  "AT_Tag_14_Yaw"
  AT_Tag_15_Yaw/1 -> Bus Creator18/12  "AT_Tag_15_Yaw"
  AT_Tag_16_Yaw/1 -> Bus Creator18/13  "AT_Tag_16_Yaw"
  AT_Tag_4_Found/1 -> Bus Creator18/14  "AT_Tag_4_Found"
  AT_Tag_5_Found/1 -> Bus Creator18/15  "AT_Tag_5_Found"
  AT_Tag_6_Found/1 -> Bus Creator18/16  "AT_Tag_6_Found"
  AT_Tag_7_Found/1 -> Bus Creator18/17  "AT_Tag_7_Found"
  AT_Tag_11_Found/1 -> Bus Creator18/18  "AT_Tag_11_Found"
  AT_Tag_12_Found/1 -> Bus Creator18/19  "AT_Tag_12_Found"
  AT_Tag_13_Found/1 -> Bus Creator18/20  "AT_Tag_13_Found"
  AT_Tag_14_Found/1 -> Bus Creator18/21  "AT_Tag_14_Found"
  AT_Tag_15_Found/1 -> Bus Creator18/22  "AT_Tag_15_Found"
  AT_Tag_16_Found/1 -> Bus Creator18/23  "AT_Tag_16_Found"
  Joystick_Left_B7/1 -> Bus Creator5/11  "Joystick_Left_B7"
  Joystick_Right_B7/1 -> Bus Creator5/19  "Joystick_Right_B7"
  Bus Selector13/20 -> Human_Input_Pre_Processing/20  "<Joystick_Right_B7>"
  Bus Selector13/12 -> Human_Input_Pre_Processing/12  "<Joystick_Left_B7>"
  Human_Input_Pre_Processing/17 -> Bus Creator24/17
  Bus Selector41/19 -> Teleop/19  "<Chain_Hook>"
  Bus Selector41/20 -> Teleop/20  "<AT_Tag_4_Yaw>"
  Bus Selector41/21 -> Teleop/21  "<AT_Tag_5_Yaw>"
  Bus Selector41/22 -> Teleop/22  "<AT_Tag_6_Yaw>"
  Bus Selector41/23 -> Teleop/23  "<AT_Tag_7_Yaw>"
  Bus Selector41/24 -> Teleop/24  "<AT_Tag_11_Yaw>"
  Bus Selector41/25 -> Teleop/25  "<AT_Tag_12_Yaw>"
  Bus Selector41/26 -> Teleop/26  "<AT_Tag_13_Yaw>"
  Bus Selector41/27 -> Teleop/27  "<AT_Tag_14_Yaw>"
  Bus Selector41/28 -> Teleop/28  "<AT_Tag_15_Yaw>"
  Bus Selector41/29 -> Teleop/29  "<AT_Tag_16_Yaw>"
  Bus Selector41/30 -> Teleop/30  "<AT_Tag_4_Found>"
  Bus Selector41/31 -> Teleop/31  "<AT_Tag_5_Found>"
  Bus Selector41/32 -> Teleop/32  "<AT_Tag_6_Found>"
  Bus Selector41/33 -> Teleop/33  "<AT_Tag_7_Found>"
  Bus Selector41/34 -> Teleop/34  "<AT_Tag_11_Found>"
  Bus Selector41/35 -> Teleop/35  "<AT_Tag_12_Found>"
  Bus Selector41/36 -> Teleop/36  "<AT_Tag_13_Found>"
  Bus Selector41/37 -> Teleop/37  "<AT_Tag_14_Found>"
  Bus Selector41/38 -> Teleop/38  "<AT_Tag_15_Found>"
  Bus Selector41/39 -> Teleop/39  "<AT_Tag_16_Found>"
  Teleop/14 -> Bus Creator2/14
  Test/14 -> Bus Creator12/14
  Bus Selector12/1 -> Test/1  "<Chain_Hook>"
  Disabled/14 -> Bus Creator4/14
  Autonomous/14 -> Bus Creator1/14
  Bus Selector15/1 -> Chain_DutyCycle/1  "<Chain_DutyCycle>"

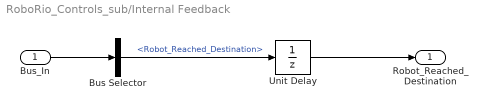
== system RoboRio_Controls_sub/Internal Feedback ==
  Bus_In : Inport
  Bus Selector : BusSelector  OutputSignals=Robot_Reached_Destination
  Unit Delay : UnitDelay  SampleTime=-1  HasFrameUpgradeWarning=on
  Robot_Reached_Destination : Outport
  wires:
  Unit Delay/1 -> Robot_Reached_Destination/1
  Bus Selector/1 -> Unit Delay/1  "<Robot_Reached_Destination>"
  Bus_In/1 -> Bus Selector/1

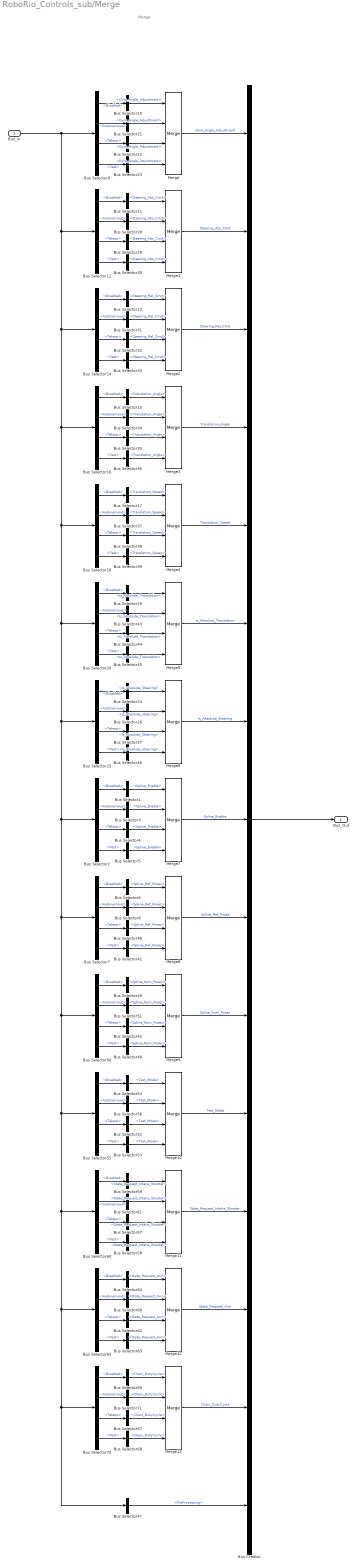
== system RoboRio_Controls_sub/Merge ==
  note: Merge
  Bus_In : Inport
  Bus Creator : BusCreator  Inputs=15
  Bus Selector{1,3..5} (4 alike) : BusSelector  OutputSignals=Spline_Enable
  Bus Selector{10,21..23} (4 alike) : BusSelector  OutputSignals=Gyro_Angle_Adjustment
  Bus Selector{11,28..30} (4 alike) : BusSelector  OutputSignals=Steering_Abs_Cmd
  Bus Selector{2,7,9,12,14,16,18,20,25,50,55,60,65,70} (14 alike) : BusSelector  OutputSignals=Disabled,Autonomous,Teleop,Test
  Bus Selector{13,31..33} (4 alike) : BusSelector  OutputSignals=Steering_Rel_Cmd
  Bus Selector{15,34..36} (4 alike) : BusSelector  OutputSignals=Translation_Angle
  Bus Selector{17,37..39} (4 alike) : BusSelector  OutputSignals=Translation_Speed
  Bus Selector{19,43..45} (4 alike) : BusSelector  OutputSignals=Is_Absolute_Translation
  Bus Selector{24,26..27,46} (4 alike) : BusSelector  OutputSignals=Is_Absolute_Steering
  Bus Selector{6,8,40..41} (4 alike) : BusSelector  OutputSignals=Spline_Ref_Poses
  Bus Selector{42,48..49,51} (4 alike) : BusSelector  OutputSignals=Spline_Num_Poses
  Bus Selector47 : BusSelector  OutputSignals=PreProcessing
  Bus Selector{52..54,56} (4 alike) : BusSelector  OutputSignals=Test_Mode
  Bus Selector{57..59,61} (4 alike) : BusSelector  OutputSignals=State_Request_Intake_Shooter
  Bus Selector{62..64,66} (4 alike) : BusSelector  OutputSignals=State_Request_Arm
  Bus Selector{67..69,71} (4 alike) : BusSelector  OutputSignals=Chain_DutyCycle
  Merge{,1..13} (14 alike) : Merge  Inputs=4
  Bus_Out : Outport
  wires:
  Merge13/1 -> Bus Creator/14  "Chain_DutyCycle"
  Bus Selector70/3 -> Bus Selector67/1  "<Teleop>"
  Bus Selector67/1 -> Merge13/3  "<Chain_DutyCycle>"
  Bus Selector71/1 -> Merge13/2  "<Chain_DutyCycle>"
  Bus Selector70/4 -> Bus Selector68/1  "<Test>"
  Bus Selector70/1 -> Bus Selector69/1  "<Disabled>"
  Bus Selector69/1 -> Merge13/1  "<Chain_DutyCycle>"
  Bus Selector68/1 -> Merge13/4  "<Chain_DutyCycle>"
  Bus Selector70/2 -> Bus Selector71/1  "<Autonomous>"
  Merge12/1 -> Bus Creator/13  "State_Request_Arm"
  Bus Selector65/2 -> Bus Selector66/1  "<Autonomous>"
  Bus Selector63/1 -> Merge12/4  "<State_Request_Arm>"
  Bus Selector64/1 -> Merge12/1  "<State_Request_Arm>"
  Bus Selector65/1 -> Bus Selector64/1  "<Disabled>"
  Bus Selector65/4 -> Bus Selector63/1  "<Test>"
  Bus Selector66/1 -> Merge12/2  "<State_Request_Arm>"
  Bus Selector62/1 -> Merge12/3  "<State_Request_Arm>"
  Bus Selector65/3 -> Bus Selector62/1  "<Teleop>"
  Merge11/1 -> Bus Creator/12  "State_Request_Intake_Shooter"
  Bus Selector60/3 -> Bus Selector57/1  "<Teleop>"
  Bus Selector57/1 -> Merge11/3  "<State_Request_Intake_Shooter>"
  Bus Selector61/1 -> Merge11/2  "<State_Request_Intake_Shooter>"
  Bus Selector60/4 -> Bus Selector58/1  "<Test>"
  Bus Selector60/1 -> Bus Selector59/1  "<Disabled>"
  Bus Selector59/1 -> Merge11/1  "<State_Request_Intake_Shooter>"
  Bus Selector58/1 -> Merge11/4  "<State_Request_Intake_Shooter>"
  Bus Selector60/2 -> Bus Selector61/1  "<Autonomous>"
  Merge10/1 -> Bus Creator/11  "Test_Mode"
  Bus Selector55/2 -> Bus Selector56/1  "<Autonomous>"
  Bus Selector53/1 -> Merge10/4  "<Test_Mode>"
  Bus Selector54/1 -> Merge10/1  "<Test_Mode>"
  Bus Selector55/1 -> Bus Selector54/1  "<Disabled>"
  Bus Selector55/4 -> Bus Selector53/1  "<Test>"
  Bus Selector56/1 -> Merge10/2  "<Test_Mode>"
  Bus Selector52/1 -> Merge10/3  "<Test_Mode>"
  Bus Selector55/3 -> Bus Selector52/1  "<Teleop>"
  Merge9/1 -> Bus Creator/10  "Spline_Num_Poses"
  Bus Selector48/1 -> Merge9/4  "<Spline_Num_Poses>"
  Bus Selector50/1 -> Bus Selector49/1  "<Disabled>"
  Bus Selector42/1 -> Merge9/3  "<Spline_Num_Poses>"
  Bus Selector49/1 -> Merge9/1  "<Spline_Num_Poses>"
  Bus Selector51/1 -> Merge9/2  "<Spline_Num_Poses>"
  Bus Selector50/4 -> Bus Selector48/1  "<Test>"
  Bus Selector50/3 -> Bus Selector42/1  "<Teleop>"
  Bus Selector50/2 -> Bus Selector51/1  "<Autonomous>"
  Merge8/1 -> Bus Creator/9  "Spline_Ref_Poses"
  Bus Selector7/2 -> Bus Selector8/1  "<Autonomous>"
  Bus Selector7/3 -> Bus Selector40/1  "<Teleop>"
  Bus Selector7/4 -> Bus Selector41/1  "<Test>"
  Bus Selector8/1 -> Merge8/2  "<Spline_Ref_Poses>"
  Bus Selector6/1 -> Merge8/1  "<Spline_Ref_Poses>"
  Bus Selector40/1 -> Merge8/3  "<Spline_Ref_Poses>"
  Bus Selector7/1 -> Bus Selector6/1  "<Disabled>"
  Bus Selector41/1 -> Merge8/4  "<Spline_Ref_Poses>"
  Merge7/1 -> Bus Creator/8  "Spline_Enable"
  Bus Selector5/1 -> Merge7/4  "<Spline_Enable>"
  Bus Selector2/1 -> Bus Selector1/1  "<Disabled>"
  Bus Selector4/1 -> Merge7/3  "<Spline_Enable>"
  Bus Selector1/1 -> Merge7/1  "<Spline_Enable>"
  Bus Selector3/1 -> Merge7/2  "<Spline_Enable>"
  Bus Selector2/4 -> Bus Selector5/1  "<Test>"
  Bus Selector2/3 -> Bus Selector4/1  "<Teleop>"
  Bus Selector2/2 -> Bus Selector3/1  "<Autonomous>"
  Bus Creator/1 -> Bus_Out/1
  Bus Selector29/1 -> Merge1/3  "<Steering_Abs_Cmd>"
  Bus Selector25/2 -> Bus Selector26/1  "<Autonomous>"
  Bus Selector25/3 -> Bus Selector27/1  "<Teleop>"
  Bus Selector14/3 -> Bus Selector32/1  "<Teleop>"
  Bus Selector16/3 -> Bus Selector35/1  "<Teleop>"
  Bus Selector16/4 -> Bus Selector36/1  "<Test>"
  Bus Selector20/1 -> Bus Selector19/1  "<Disabled>"
  Merge1/1 -> Bus Creator/2  "Steering_Abs_Cmd"
  Bus Selector34/1 -> Merge3/2  "<Translation_Angle>"
  Merge/1 -> Bus Creator/1  "Gyro_Angle_Adjustment"
  Bus Selector17/1 -> Merge4/1  "<Translation_Speed>"
  Bus Selector15/1 -> Merge3/1  "<Translation_Angle>"
  Bus Selector21/1 -> Merge/2  "<Gyro_Angle_Adjustment>"
  Bus Selector9/3 -> Bus Selector22/1  "<Teleop>"
  Bus Selector20/2 -> Bus Selector43/1  "<Autonomous>"
  Bus Selector14/1 -> Bus Selector13/1  "<Disabled>"
  Bus Selector23/1 -> Merge/4  "<Gyro_Angle_Adjustment>"
  Bus Selector20/4 -> Bus Selector45/1  "<Test>"
  Bus Selector10/1 -> Merge/1  "<Gyro_Angle_Adjustment>"
  Merge5/1 -> Bus Creator/6  "Is_Absolute_Translation"
  Bus Selector36/1 -> Merge3/4  "<Translation_Angle>"
  Bus Selector47/1 -> Bus Creator/15  "<PreProcessing>"
  Bus Selector12/1 -> Bus Selector11/1  "<Disabled>"
  Bus Selector16/2 -> Bus Selector34/1  "<Autonomous>"
  Bus Selector22/1 -> Merge/3  "<Gyro_Angle_Adjustment>"
  Bus Selector37/1 -> Merge4/2  "<Translation_Speed>"
  Bus Selector25/4 -> Bus Selector46/1  "<Test>"
  Bus Selector18/3 -> Bus Selector38/1  "<Teleop>"
  Bus Selector20/3 -> Bus Selector44/1  "<Teleop>"
  Bus Selector39/1 -> Merge4/4  "<Translation_Speed>"
  Bus Selector16/1 -> Bus Selector15/1  "<Disabled>"
  Bus Selector13/1 -> Merge2/1  "<Steering_Rel_Cmd>"
  Bus Selector30/1 -> Merge1/4  "<Steering_Abs_Cmd>"
  Bus Selector26/1 -> Merge6/2  "<Is_Absolute_Steering>"
  Merge6/1 -> Bus Creator/7  "Is_Absolute_Steering"
  Bus Selector18/1 -> Bus Selector17/1  "<Disabled>"
  Bus Selector45/1 -> Merge5/4  "<Is_Absolute_Translation>"
  Bus Selector12/3 -> Bus Selector29/1  "<Teleop>"
  Bus Selector18/2 -> Bus Selector37/1  "<Autonomous>"
  Bus Selector43/1 -> Merge5/2  "<Is_Absolute_Translation>"
  Bus Selector19/1 -> Merge5/1  "<Is_Absolute_Translation>"
  Bus Selector35/1 -> Merge3/3  "<Translation_Angle>"
  Merge3/1 -> Bus Creator/4  "Translation_Angle"
  Bus Selector28/1 -> Merge1/2  "<Steering_Abs_Cmd>"
  Bus Selector14/2 -> Bus Selector31/1  "<Autonomous>"
  Bus Selector32/1 -> Merge2/3  "<Steering_Rel_Cmd>"
  Merge4/1 -> Bus Creator/5  "Translation_Speed"
  Bus Selector12/2 -> Bus Selector28/1  "<Autonomous>"
  Bus Selector14/4 -> Bus Selector33/1  "<Test>"
  Bus Selector44/1 -> Merge5/3  "<Is_Absolute_Translation>"
  Bus Selector24/1 -> Merge6/1  "<Is_Absolute_Steering>"
  Bus Selector11/1 -> Merge1/1  "<Steering_Abs_Cmd>"
  Bus Selector9/2 -> Bus Selector21/1  "<Autonomous>"
  Bus Selector31/1 -> Merge2/2  "<Steering_Rel_Cmd>"
  Bus Selector27/1 -> Merge6/3  "<Is_Absolute_Steering>"
  Bus Selector25/1 -> Bus Selector24/1  "<Disabled>"
  Bus Selector18/4 -> Bus Selector39/1  "<Test>"
  Bus Selector46/1 -> Merge6/4  "<Is_Absolute_Steering>"
  Bus Selector9/4 -> Bus Selector23/1  "<Test>"
  Bus Selector38/1 -> Merge4/3  "<Translation_Speed>"
  Bus Selector33/1 -> Merge2/4  "<Steering_Rel_Cmd>"
  Bus Selector9/1 -> Bus Selector10/1  "<Disabled>"
  Bus_In/1 -> Bus Selector9/1, Bus Selector12/1, Bus Selector14/1, Bus Selector16/1, Bus Selector18/1, Bus Selector20/1, Bus Selector25/1, Bus Selector47/1, Bus Selector70/1, Bus Selector65/1, Bus Selector60/1, Bus Selector55/1, Bus Selector50/1, Bus Selector7/1, Bus Selector2/1
  Bus Selector12/4 -> Bus Selector30/1  "<Test>"
  Merge2/1 -> Bus Creator/3  "Steering_Rel_Cmd"
